simulink model "Junctions1"  (Simulink 9.0)
settings: Solver=FixedStepDiscrete  StartTime=0.0  StopTime=10.0  RelTol=1e-3  EnableMultiTasking=on
settings Model: SuppressorTable=22 serialization::archive 11 0 6 0 0 0 0 0  Creator=scaife  LastModifiedBy=hbourbou  ExtModeAutoUpdateStatusClock=off
settings DataIOCC: LimitDataPoints=on  SignalLoggingSaveFormat=ModelDataLogs  SignalLoggingName=sigsOut
settings DebuggingCC: SaveWithParameterizedLinksMsg=none  SignalResolutionControl=TryResolveAllWithWarning  MultiTaskDSMMsg=warning  MultiTaskCondExecSysMsg=none
settings HardwareCC: TargetUnknown=on
settings SFSimCC: SimParseCustomCode=off
settings GRTTargetCC: GeneratePreprocessorConditionals=Disable all  CombineOutputUpdateFcns=off  GRTInterface=on

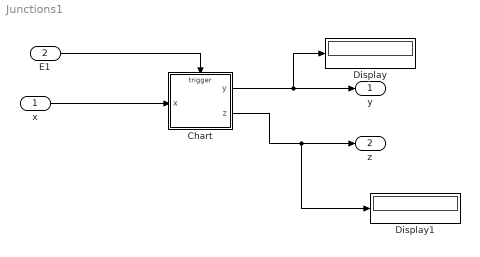
== system Junctions1 ==
  x : Inport
  E1 : Inport  Port=2
  Chart : Stateflow chart  TreatAsAtomicUnit=on
  Display : Display
  Display1 : Display
  y : Outport
  z : Outport  Port=2
  wires:
  x/1 -> Chart/1(x)
  E1/1 -> Chart/Trigger
  Chart/1(y) -> Display/1, y/1
  Chart/2(z) -> Display1/1, z/1

== stateflow chart Chart ==
  state A
    ex : y=y.*2
  state C
  state B
  B -> A : [x>3]
  (default) -> A
  C -> A : [x>3]
  A -> (junction 10) : E1[x>0]{y = y + 1;z = z + 2}
  (junction 10) -> C [order 2] : [x<2]{y = y + 1;z = z + 1}
  (junction 10) -> B [order 1] : [x>=2]{y = y + 2;z = z + 1}
  data: x input int32; y output int32 =int32(1); z output int32 =int32(2)
  events: E1 input EITHER_EDGE_EVENT
